simulink model "readFromMat"  (R2015a)
settings: Solver=ode3  StartTime=0.0  StopTime=100  FixedStep=0.01  RelTol=1e-3
settings Model: Creator=shawn  LastModifiedBy=shawn

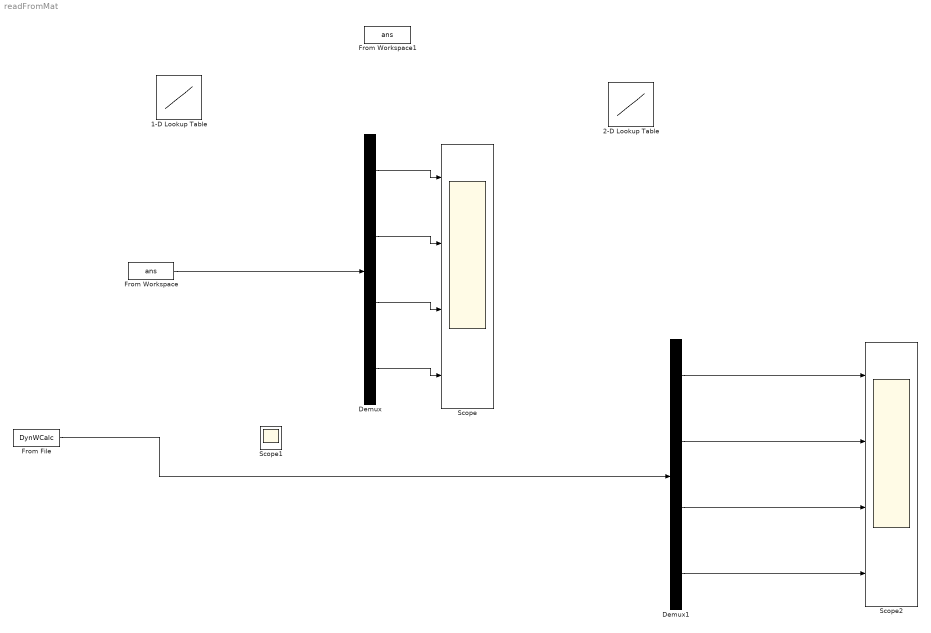
== system readFromMat ==
  1-D Lookup Table : Lookup_n-D  NumberOfTableDimensions=1  BreakpointsForDimension1=[-5:5]  Table=tanh([-5:5])  InternalRulePriority=Speed  RndMeth=Simplest  InputSameDT=on
  2-D Lookup Table : Lookup_n-D  BreakpointsForDimension1=[1:3]  BreakpointsForDimension2=[1:3]  InternalRulePriority=Speed  RndMeth=Simplest  InputSameDT=on
  Demux : Demux
  Demux1 : Demux
  From Workspace : FromWorkspace  VariableName=ans  SampleTime=0
  From Workspace1 : FromWorkspace  VariableName=ans  SampleTime=0
  From File : FromFile  FileName=DynWCalc  SampleTime=0
  Scope : Scope  NumInputPorts=4
      settings: YMin=-5~-5~-5~-5  YMax=5~5~5~5
  Scope1 : Scope
  Scope2 : Scope  NumInputPorts=4
      settings: YMin=-5~-5~-5~-5  YMax=5~5~5~5  SaveName=ScopeData2
  wires:
  From Workspace/1 -> Demux/1
  Demux/2 -> Scope/2
  Demux/1 -> Scope/1
  Demux/3 -> Scope/3
  Demux/4 -> Scope/4
  From File/1 -> Demux1/1
  Demux1/3 -> Scope2/3
  Demux1/4 -> Scope2/4
  Demux1/2 -> Scope2/2
  Demux1/1 -> Scope2/1
